simulink library "SOEM_EtherCAT_Lib"  (R2017b)
settings: Solver=ode45  StartTime=0.0  StopTime=10.0  RelTol=1e-3  EnableMultiTasking=on
settings Model: Creator=RecSet  LastModifiedBy=root
settings DataIOCC: LimitDataPoints=on  SaveFormat=Array
settings OptimizationCC: LifeSpan=inf
settings DebuggingCC: SolverPrmCheckMsg=warning  SFUnexpectedBacktrackingDiag=warning  SFNoUnconditionalDefaultTransitionDiag=warning  SFExecutionAtInitializationDiag=none
settings HardwareCC: ProdBitPerPointer=32  ProdBitPerSizeT=32  ProdBitPerPtrDiffT=32  ProdLargestAtomicFloat=None  ProdIntDivRoundTo=Undefined  ProdEndianess=Unspecified  ProdWordSize=32  ProdHWDeviceType=32-bit Generic
settings ModelReferenceCC: PropagateSignalLabelsOutOfModel=off
settings CodeAppCC: StateflowObjectComments=on
settings GRTTargetCC: TargetLangStandard=C89/C90 (ANSI)  GeneratePreprocessorConditionals=Disable all
settings ConfigComp: CovMetricSettings=dw  CovHtmlReporting=on  CovSaveCumulativeToWorkspaceVar=on  CovSaveSingleToWorkspaceVar=on  CovExternalEMLEnable=off  CovSFcnEnable=off

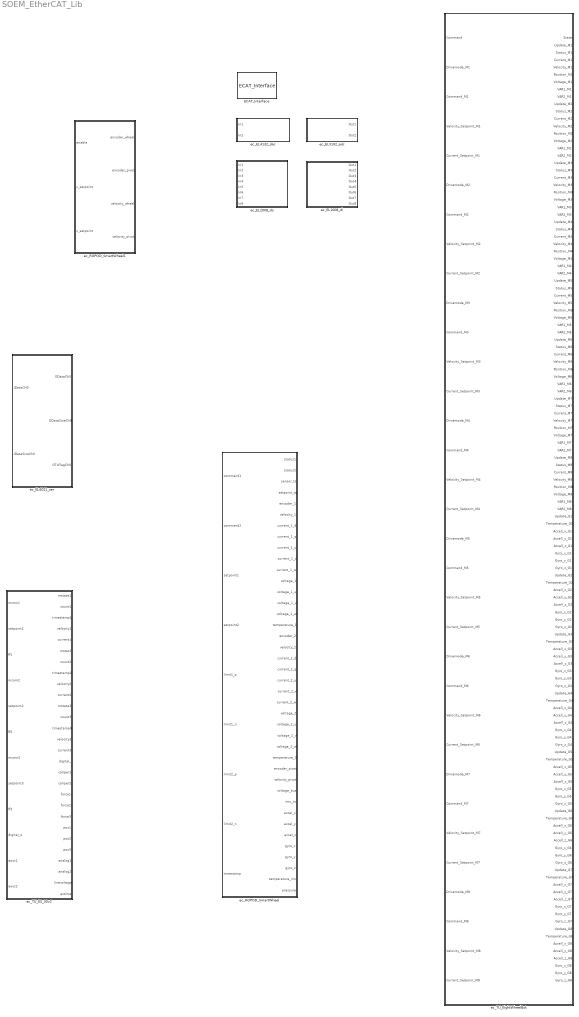
== system SOEM_EtherCAT_Lib ==
  ECAT_Interface : S-Function  Priority=0  StopFcn=|  FunctionName=ECAT_Interface  Parameters=IFINTERFACE,TS  SFunctionDeploymentMode=off  EnableBusSupport=off  mask{IFINTERFACE=eth0, TS=1/1000}
      | t_ = timer('Name','DLL_Unload_timer',...
      |             'ExecutionMode','singleShot',...
      |             'StartDelay',2,...
      |             'StopFcn','try;delete(t_);clear(''t_'');catch;disp(''Unloading DLL Failed!'');end;',...
      |             'TimerFcn','clear mex;'); 
      | start(t_);
      mask prompts: TS "Block sample time [s]"
      mask Callback IFINTERFACE:
      | VAR = get_param(gcb, 'IFINTERFACE');
      | if ~isnan(str2double(VAR))
      |     errordlg('Enter a string!');
      |     set_param(gcb, 'IFINTERFACE', '\Device\NPF_{$KEY}');
      | end
      mask DialogControl ParameterGroupVar Prompt: String with network device this block needs to use
  ec_EL1008_di : Subsystem  mask(EL1008 di){LINKID=1}
      mask prompts: LINKID "Enter link id (>0)"
  ec_EL2008_do : Subsystem  mask(EL2008 do){LINKID=1}
      mask prompts: LINKID "Enter link id (>0)"
  ec_EL3102_adc : Subsystem  mask(EL3102 adc){LINKID=1}
      mask prompts: LINKID "Enter link id (>0)"
  ec_EL4132_dac : Subsystem  mask(EL4132 dac){LINKID=1}
      mask prompts: LINKID "Enter link id (>0)"
  ec_EL6021_ser : Subsystem  mask{link_id=1}
      mask prompts: link_id "Link id (>0)"
  ec_ROPOD_SmartWheel : Subsystem  mask{link_id=1}
      mask prompts: link_id "Link id (>0)"
  ec_ROPOD_SmartWheel1 : Subsystem  mask{link_id=1}
      mask prompts: link_id "Link id (>0)"
  ec_TU_ES_30v2 : Subsystem  mask{link_id=1}
      mask prompts: link_id "Link id (>0)"
  ec_TU_EightWheelBot : Subsystem  mask(TU_EightWheelBot){LINKID=1}
      mask prompts: LINKID "Enter link id (>0)"

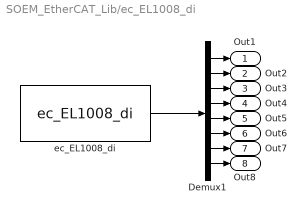
== system SOEM_EtherCAT_Lib/ec_EL1008_di ==
  Demux1 : Demux  Outputs=8
  ec_EL1008_di : S-Function  Priority=1  FunctionName=ec_EL1008_di  Parameters=LINKID  SFunctionDeploymentMode=off  EnableBusSupport=off
  Out1 : Outport
  Out2 : Outport  Port=2
  Out3 : Outport  Port=3
  Out4 : Outport  Port=4
  Out5 : Outport  Port=5
  Out6 : Outport  Port=6
  Out7 : Outport  Port=7
  Out8 : Outport  Port=8
  wires:
  Demux1/3 -> Out3/1
  Demux1/5 -> Out5/1
  Demux1/8 -> Out8/1
  Demux1/2 -> Out2/1
  Demux1/4 -> Out4/1
  Demux1/1 -> Out1/1
  Demux1/6 -> Out6/1
  Demux1/7 -> Out7/1
  ec_EL1008_di/1 -> Demux1/1

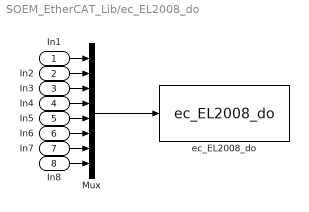
== system SOEM_EtherCAT_Lib/ec_EL2008_do ==
  In1 : Inport
  In2 : Inport  Port=2
  In3 : Inport  Port=3
  In4 : Inport  Port=4
  In5 : Inport  Port=5
  In6 : Inport  Port=6
  In7 : Inport  Port=7
  In8 : Inport  Port=8
  Mux : Mux  Inputs=8
  ec_EL2008_do : S-Function  Priority=1  FunctionName=ec_EL2008_do  Parameters=LINKID  SFunctionDeploymentMode=off  EnableBusSupport=off
  wires:
  In8/1 -> Mux/8
  In6/1 -> Mux/6
  In1/1 -> Mux/1
  In2/1 -> Mux/2
  In7/1 -> Mux/7
  In3/1 -> Mux/3
  In4/1 -> Mux/4
  In5/1 -> Mux/5
  Mux/1 -> ec_EL2008_do/1

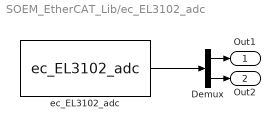
== system SOEM_EtherCAT_Lib/ec_EL3102_adc ==
  Demux : Demux  Outputs=2
  ec_EL3102_adc : S-Function  Priority=1  FunctionName=ec_EL3102_adc  Parameters=LINKID  SFunctionDeploymentMode=off  EnableBusSupport=off
  Out1 : Outport
  Out2 : Outport  Port=2
  wires:
  Demux/1 -> Out1/1
  Demux/2 -> Out2/1
  ec_EL3102_adc/1 -> Demux/1

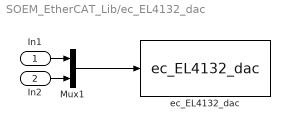
== system SOEM_EtherCAT_Lib/ec_EL4132_dac ==
  In1 : Inport
  In2 : Inport  Port=2
  Mux1 : Mux  Inputs=2
  ec_EL4132_dac : S-Function  Priority=1  FunctionName=ec_EL4132_dac  Parameters=LINKID  SFunctionDeploymentMode=off  EnableBusSupport=off
  wires:
  Mux1/1 -> ec_EL4132_dac/1
  In2/1 -> Mux1/2
  In1/1 -> Mux1/1

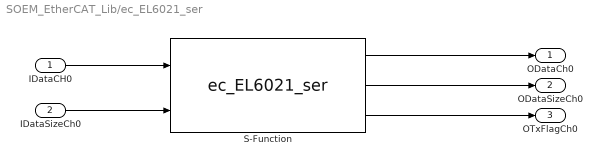
== system SOEM_EtherCAT_Lib/ec_EL6021_ser ==
  IDataCH0 : Inport
  IDataSizeCh0 : Inport  Port=2
  S-Function : S-Function  FunctionName=ec_EL6021_ser  Parameters=link_id  SFunctionDeploymentMode=off  EnableBusSupport=off  mask{link_id=link_id}
      mask prompts: link_id "Link id (start from 1)"
  ODataCh0 : Outport
  ODataSizeCh0 : Outport  Port=2
  OTxFlagCh0 : Outport  Port=3
  wires:
  IDataCH0/1 -> S-Function/1
  IDataSizeCh0/1 -> S-Function/2
  S-Function/1 -> ODataCh0/1
  S-Function/2 -> ODataSizeCh0/1
  S-Function/3 -> OTxFlagCh0/1

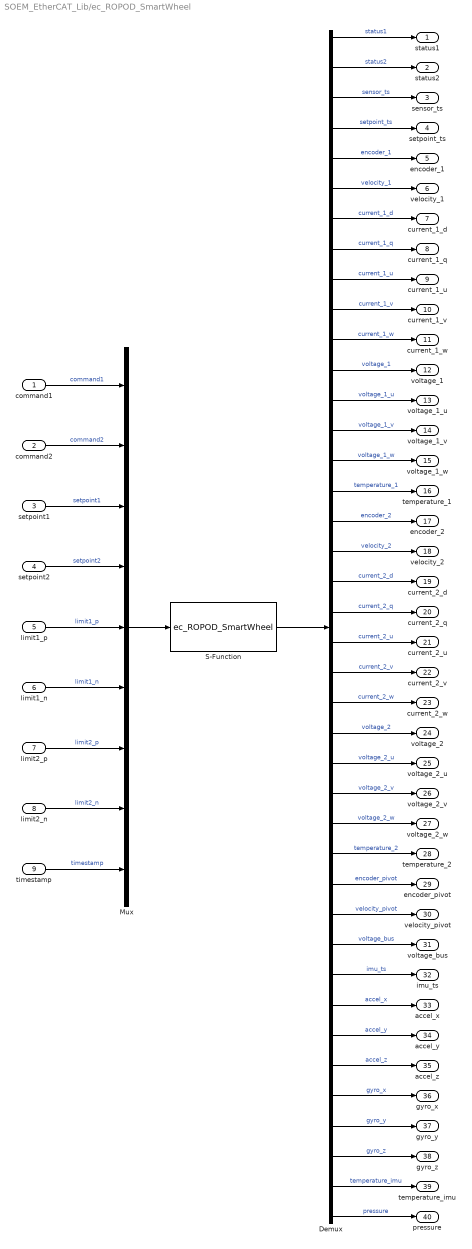
== system SOEM_EtherCAT_Lib/ec_ROPOD_SmartWheel ==
  command1 : Inport
  command2 : Inport  Port=2
  setpoint1 : Inport  Port=3
  setpoint2 : Inport  Port=4
  limit1_p : Inport  Port=5
  limit1_n : Inport  Port=6
  limit2_p : Inport  Port=7
  limit2_n : Inport  Port=8
  timestamp : Inport  Port=9
  Demux : Demux  Outputs=40
  Mux : Mux  Inputs=9
  S-Function : S-Function  FunctionName=ec_ROPOD_SmartWheel  Parameters=link_id  SFunctionDeploymentMode=off  EnableBusSupport=off  mask{link_id=link_id}
      mask prompts: link_id "Link id (start from 1)"
  status1 : Outport
  status2 : Outport  Port=2
  sensor_ts : Outport  Port=3
  setpoint_ts : Outport  Port=4
  encoder_1 : Outport  Port=5
  velocity_1 : Outport  Port=6
  current_1_d : Outport  Port=7
  current_1_q : Outport  Port=8
  current_1_u : Outport  Port=9
  current_1_v : Outport  Port=10
  current_1_w : Outport  Port=11
  voltage_1 : Outport  Port=12
  voltage_1_u : Outport  Port=13
  voltage_1_v : Outport  Port=14
  voltage_1_w : Outport  Port=15
  temperature_1 : Outport  Port=16
  encoder_2 : Outport  Port=17
  velocity_2 : Outport  Port=18
  current_2_d : Outport  Port=19
  current_2_q : Outport  Port=20
  current_2_u : Outport  Port=21
  current_2_v : Outport  Port=22
  current_2_w : Outport  Port=23
  voltage_2 : Outport  Port=24
  voltage_2_u : Outport  Port=25
  voltage_2_v : Outport  Port=26
  voltage_2_w : Outport  Port=27
  temperature_2 : Outport  Port=28
  encoder_pivot : Outport  Port=29
  velocity_pivot : Outport  Port=30
  voltage_bus : Outport  Port=31
  imu_ts : Outport  Port=32
  accel_x : Outport  Port=33
  accel_y : Outport  Port=34
  accel_z : Outport  Port=35
  gyro_x : Outport  Port=36
  gyro_y : Outport  Port=37
  gyro_z : Outport  Port=38
  temperature_imu : Outport  Port=39
  pressure : Outport  Port=40
  wires:
  Mux/1 -> S-Function/1
  timestamp/1 -> Mux/9  "timestamp"
  limit2_n/1 -> Mux/8  "limit2_n"
  limit2_p/1 -> Mux/7  "limit2_p"
  Demux/28 -> temperature_2/1  "temperature_2"
  Demux/27 -> voltage_2_w/1  "voltage_2_w"
  Demux/26 -> voltage_2_v/1  "voltage_2_v"
  Demux/25 -> voltage_2_u/1  "voltage_2_u"
  Demux/24 -> voltage_2/1  "voltage_2"
  Demux/23 -> current_2_w/1  "current_2_w"
  Demux/22 -> current_2_v/1  "current_2_v"
  Demux/21 -> current_2_u/1  "current_2_u"
  Demux/20 -> current_2_q/1  "current_2_q"
  Demux/19 -> current_2_d/1  "current_2_d"
  Demux/18 -> velocity_2/1  "velocity_2"
  Demux/17 -> encoder_2/1  "encoder_2"
  Demux/16 -> temperature_1/1  "temperature_1"
  Demux/15 -> voltage_1_w/1  "voltage_1_w"
  Demux/14 -> voltage_1_v/1  "voltage_1_v"
  Demux/13 -> voltage_1_u/1  "voltage_1_u"
  Demux/12 -> voltage_1/1  "voltage_1"
  Demux/11 -> current_1_w/1  "current_1_w"
  Demux/10 -> current_1_v/1  "current_1_v"
  Demux/9 -> current_1_u/1  "current_1_u"
  Demux/8 -> current_1_q/1  "current_1_q"
  Demux/7 -> current_1_d/1  "current_1_d"
  Demux/6 -> velocity_1/1  "velocity_1"
  Demux/5 -> encoder_1/1  "encoder_1"
  Demux/4 -> setpoint_ts/1  "setpoint_ts"
  Demux/3 -> sensor_ts/1  "sensor_ts"
  Demux/2 -> status2/1  "status2"
  limit1_n/1 -> Mux/6  "limit1_n"
  limit1_p/1 -> Mux/5  "limit1_p"
  setpoint2/1 -> Mux/4  "setpoint2"
  setpoint1/1 -> Mux/3  "setpoint1"
  Demux/1 -> status1/1  "status1"
  command2/1 -> Mux/2  "command2"
  command1/1 -> Mux/1  "command1"
  S-Function/1 -> Demux/1
  Demux/29 -> encoder_pivot/1  "encoder_pivot"
  Demux/30 -> velocity_pivot/1  "velocity_pivot"
  Demux/31 -> voltage_bus/1  "voltage_bus"
  Demux/32 -> imu_ts/1  "imu_ts"
  Demux/33 -> accel_x/1  "accel_x"
  Demux/34 -> accel_y/1  "accel_y"
  Demux/35 -> accel_z/1  "accel_z"
  Demux/36 -> gyro_x/1  "gyro_x"
  Demux/37 -> gyro_y/1  "gyro_y"
  Demux/38 -> gyro_z/1  "gyro_z"
  Demux/39 -> temperature_imu/1  "temperature_imu"
  Demux/40 -> pressure/1  "pressure"

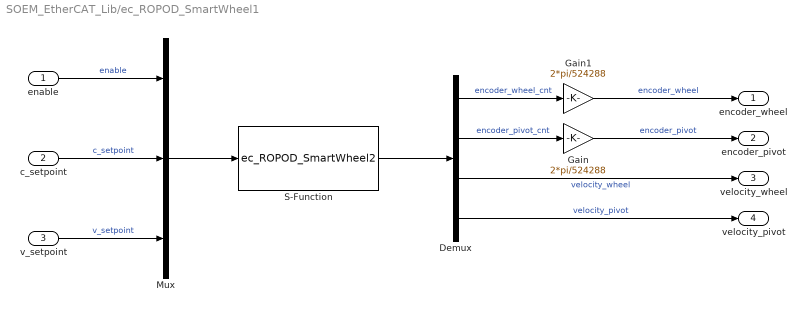
== system SOEM_EtherCAT_Lib/ec_ROPOD_SmartWheel1 ==
  enable : Inport
  c_setpoint : Inport  Port=2
  v_setpoint : Inport  Port=3
  Demux : Demux
  Gain : Gain  Gain=2*pi/524288
  Gain1 : Gain  Gain=2*pi/524288
  Mux : Mux  Inputs=3
  S-Function : S-Function  FunctionName=ec_ROPOD_SmartWheel2  Parameters=link_id  SFunctionDeploymentMode=off  EnableBusSupport=off  mask{link_id=link_id}
      mask prompts: link_id "Link id (start from 1)"
  encoder_wheel : Outport
  encoder_pivot : Outport  Port=2
  velocity_wheel : Outport  Port=3
  velocity_pivot : Outport  Port=4
  wires:
  Mux/1 -> S-Function/1
  Demux/4 -> velocity_pivot/1  "velocity_pivot"
  Demux/3 -> velocity_wheel/1  "velocity_wheel"
  Demux/2 -> Gain/1  "encoder_pivot_cnt"
  v_setpoint/1 -> Mux/3  "v_setpoint"
  Demux/1 -> Gain1/1  "encoder_wheel_cnt"
  c_setpoint/1 -> Mux/2  "c_setpoint"
  enable/1 -> Mux/1  "enable"
  S-Function/1 -> Demux/1
  Gain/1 -> encoder_pivot/1  "encoder_pivot"
  Gain1/1 -> encoder_wheel/1  "encoder_wheel"

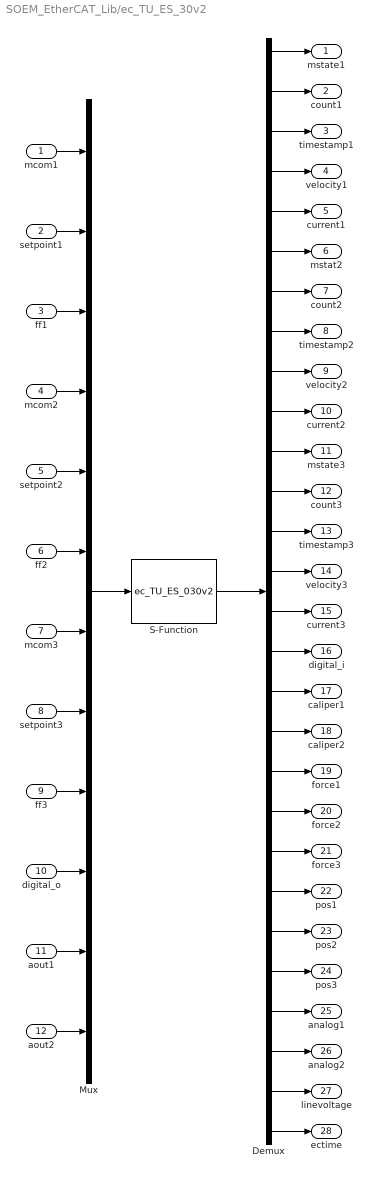
== system SOEM_EtherCAT_Lib/ec_TU_ES_30v2 ==
  mcom1 : Inport
  setpoint1 : Inport  Port=2
  ff1 : Inport  Port=3
  mcom2 : Inport  Port=4
  setpoint2 : Inport  Port=5
  ff2 : Inport  Port=6
  mcom3 : Inport  Port=7
  setpoint3 : Inport  Port=8
  ff3 : Inport  Port=9
  digital_o : Inport  Port=10
  aout1 : Inport  Port=11
  aout2 : Inport  Port=12
  Demux : Demux  Outputs=28
  Mux : Mux  Inputs=12
  S-Function : S-Function  FunctionName=ec_TU_ES_030v2  Parameters=link_id  SFunctionDeploymentMode=off  EnableBusSupport=off  mask{link_id=link_id}
      mask prompts: link_id "Link id (start from 1)"
  mstate1 : Outport
  count1 : Outport  Port=2
  timestamp1 : Outport  Port=3
  velocity1 : Outport  Port=4
  current1 : Outport  Port=5
  mstat2 : Outport  Port=6
  count2 : Outport  Port=7
  timestamp2 : Outport  Port=8
  velocity2 : Outport  Port=9
  current2 : Outport  Port=10
  mstate3 : Outport  Port=11
  count3 : Outport  Port=12
  timestamp3 : Outport  Port=13
  velocity3 : Outport  Port=14
  current3 : Outport  Port=15
  digital_i : Outport  Port=16
  caliper1 : Outport  Port=17
  caliper2 : Outport  Port=18
  force1 : Outport  Port=19
  force2 : Outport  Port=20
  force3 : Outport  Port=21
  pos1 : Outport  Port=22
  pos2 : Outport  Port=23
  pos3 : Outport  Port=24
  analog1 : Outport  Port=25
  analog2 : Outport  Port=26
  linevoltage : Outport  Port=27
  ectime : Outport  Port=28
  wires:
  S-Function/1 -> Demux/1
  mcom1/1 -> Mux/1
  setpoint1/1 -> Mux/2
  Demux/1 -> mstate1/1
  ff1/1 -> Mux/3
  mcom2/1 -> Mux/4
  setpoint2/1 -> Mux/5
  ff2/1 -> Mux/6
  Demux/2 -> count1/1
  Demux/3 -> timestamp1/1
  Demux/4 -> velocity1/1
  Demux/5 -> current1/1
  Demux/6 -> mstat2/1
  Demux/7 -> count2/1
  Demux/8 -> timestamp2/1
  Demux/9 -> velocity2/1
  Demux/10 -> current2/1
  Demux/11 -> mstate3/1
  Demux/12 -> count3/1
  Demux/13 -> timestamp3/1
  Demux/14 -> velocity3/1
  Demux/15 -> current3/1
  Demux/16 -> digital_i/1
  Demux/17 -> caliper1/1
  Demux/18 -> caliper2/1
  Demux/19 -> force1/1
  Demux/20 -> force2/1
  Demux/21 -> force3/1
  Demux/22 -> pos1/1
  Demux/23 -> pos2/1
  Demux/24 -> pos3/1
  Demux/25 -> analog1/1
  Demux/26 -> analog2/1
  Demux/27 -> linevoltage/1
  Demux/28 -> ectime/1
  mcom3/1 -> Mux/7
  setpoint3/1 -> Mux/8
  ff3/1 -> Mux/9
  digital_o/1 -> Mux/10
  aout1/1 -> Mux/11
  aout2/1 -> Mux/12
  Mux/1 -> S-Function/1

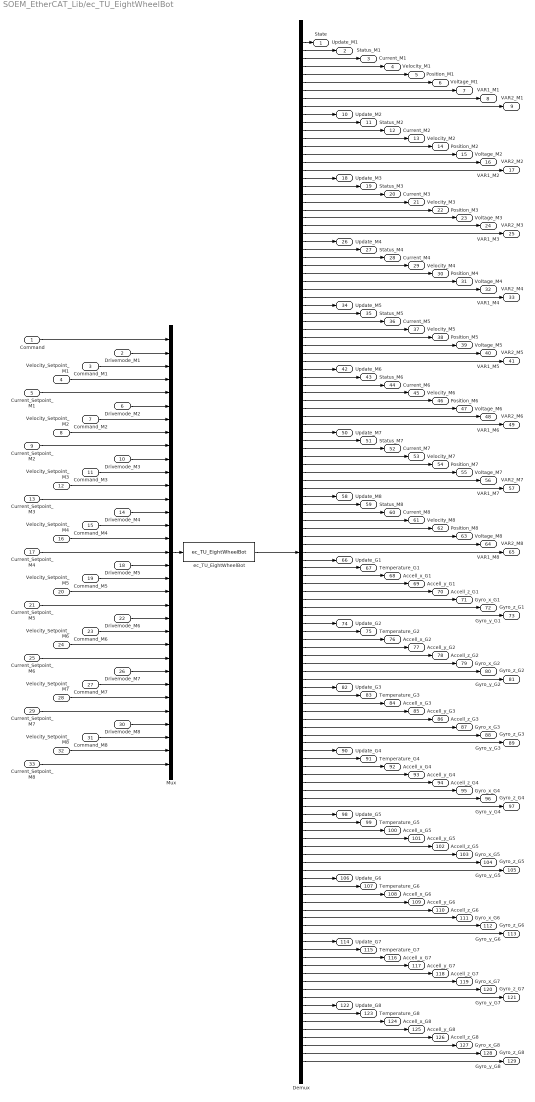
== system SOEM_EtherCAT_Lib/ec_TU_EightWheelBot ==
  Command : Inport
  Drivemode_M1 : Inport  Port=2
  Command_M1 : Inport  Port=3
  Velocity_Setpoint_M1 : Inport  Port=4
  Current_Setpoint_M1 : Inport  Port=5
  Drivemode_M2 : Inport  Port=6
  Command_M2 : Inport  Port=7
  Velocity_Setpoint_M2 : Inport  Port=8
  Current_Setpoint_M2 : Inport  Port=9
  Drivemode_M3 : Inport  Port=10
  Command_M3 : Inport  Port=11
  Velocity_Setpoint_M3 : Inport  Port=12
  Current_Setpoint_M3 : Inport  Port=13
  Drivemode_M4 : Inport  Port=14
  Command_M4 : Inport  Port=15
  Velocity_Setpoint_M4 : Inport  Port=16
  Current_Setpoint_M4 : Inport  Port=17
  Drivemode_M5 : Inport  Port=18
  Command_M5 : Inport  Port=19
  Velocity_Setpoint_M5 : Inport  Port=20
  Current_Setpoint_M5 : Inport  Port=21
  Drivemode_M6 : Inport  Port=22
  Command_M6 : Inport  Port=23
  Velocity_Setpoint_M6 : Inport  Port=24
  Current_Setpoint_M6 : Inport  Port=25
  Drivemode_M7 : Inport  Port=26
  Command_M7 : Inport  Port=27
  Velocity_Setpoint_M7 : Inport  Port=28
  Current_Setpoint_M7 : Inport  Port=29
  Drivemode_M8 : Inport  Port=30
  Command_M8 : Inport  Port=31
  Velocity_Setpoint_M8 : Inport  Port=32
  Current_Setpoint_M8 : Inport  Port=33
  Demux : Demux  Outputs=129
  Mux : Mux  Inputs=33
  ec_TU_EightWheelBot : S-Function  FunctionName=ec_TU_EightWheelBot  Parameters=LINKID  SFunctionDeploymentMode=off  EnableBusSupport=off
  State : Outport
  Update_M1 : Outport  Port=2
  Status_M1 : Outport  Port=3
  Current_M1 : Outport  Port=4
  Velocity_M1 : Outport  Port=5
  Position_M1 : Outport  Port=6
  Voltage_M1 : Outport  Port=7
  VAR1_M1 : Outport  Port=8
  VAR2_M1 : Outport  Port=9
  Update_M2 : Outport  Port=10
  Status_M2 : Outport  Port=11
  Current_M2 : Outport  Port=12
  Velocity_M2 : Outport  Port=13
  Position_M2 : Outport  Port=14
  Voltage_M2 : Outport  Port=15
  VAR1_M2 : Outport  Port=16
  VAR2_M2 : Outport  Port=17
  Update_M3 : Outport  Port=18
  Status_M3 : Outport  Port=19
  Current_M3 : Outport  Port=20
  Velocity_M3 : Outport  Port=21
  Position_M3 : Outport  Port=22
  Voltage_M3 : Outport  Port=23
  VAR1_M3 : Outport  Port=24
  VAR2_M3 : Outport  Port=25
  Update_M4 : Outport  Port=26
  Status_M4 : Outport  Port=27
  Current_M4 : Outport  Port=28
  Velocity_M4 : Outport  Port=29
  Position_M4 : Outport  Port=30
  Voltage_M4 : Outport  Port=31
  VAR1_M4 : Outport  Port=32
  VAR2_M4 : Outport  Port=33
  Update_M5 : Outport  Port=34
  Status_M5 : Outport  Port=35
  Current_M5 : Outport  Port=36
  Velocity_M5 : Outport  Port=37
  Position_M5 : Outport  Port=38
  Voltage_M5 : Outport  Port=39
  VAR1_M5 : Outport  Port=40
  VAR2_M5 : Outport  Port=41
  Update_M6 : Outport  Port=42
  Status_M6 : Outport  Port=43
  Current_M6 : Outport  Port=44
  Velocity_M6 : Outport  Port=45
  Position_M6 : Outport  Port=46
  Voltage_M6 : Outport  Port=47
  VAR1_M6 : Outport  Port=48
  VAR2_M6 : Outport  Port=49
  Update_M7 : Outport  Port=50
  Status_M7 : Outport  Port=51
  Current_M7 : Outport  Port=52
  Velocity_M7 : Outport  Port=53
  Position_M7 : Outport  Port=54
  Voltage_M7 : Outport  Port=55
  VAR1_M7 : Outport  Port=56
  VAR2_M7 : Outport  Port=57
  Update_M8 : Outport  Port=58
  Status_M8 : Outport  Port=59
  Current_M8 : Outport  Port=60
  Velocity_M8 : Outport  Port=61
  Position_M8 : Outport  Port=62
  Voltage_M8 : Outport  Port=63
  VAR1_M8 : Outport  Port=64
  VAR2_M8 : Outport  Port=65
  Update_G1 : Outport  Port=66
  Temperature_G1 : Outport  Port=67
  Accell_x_G1 : Outport  Port=68
  Accell_y_G1 : Outport  Port=69
  Accell_z_G1 : Outport  Port=70
  Gyro_x_G1 : Outport  Port=71
  Gyro_y_G1 : Outport  Port=72
  Gyro_z_G1 : Outport  Port=73
  Update_G2 : Outport  Port=74
  Temperature_G2 : Outport  Port=75
  Accell_x_G2 : Outport  Port=76
  Accell_y_G2 : Outport  Port=77
  Accell_z_G2 : Outport  Port=78
  Gyro_x_G2 : Outport  Port=79
  Gyro_y_G2 : Outport  Port=80
  Gyro_z_G2 : Outport  Port=81
  Update_G3 : Outport  Port=82
  Temperature_G3 : Outport  Port=83
  Accell_x_G3 : Outport  Port=84
  Accell_y_G3 : Outport  Port=85
  Accell_z_G3 : Outport  Port=86
  Gyro_x_G3 : Outport  Port=87
  Gyro_y_G3 : Outport  Port=88
  Gyro_z_G3 : Outport  Port=89
  Update_G4 : Outport  Port=90
  Temperature_G4 : Outport  Port=91
  Accell_x_G4 : Outport  Port=92
  Accell_y_G4 : Outport  Port=93
  Accell_z_G4 : Outport  Port=94
  Gyro_x_G4 : Outport  Port=95
  Gyro_y_G4 : Outport  Port=96
  Gyro_z_G4 : Outport  Port=97
  Update_G5 : Outport  Port=98
  Temperature_G5 : Outport  Port=99
  Accell_x_G5 : Outport  Port=100
  Accell_y_G5 : Outport  Port=101
  Accell_z_G5 : Outport  Port=102
  Gyro_x_G5 : Outport  Port=103
  Gyro_y_G5 : Outport  Port=104
  Gyro_z_G5 : Outport  Port=105
  Update_G6 : Outport  Port=106
  Temperature_G6 : Outport  Port=107
  Accell_x_G6 : Outport  Port=108
  Accell_y_G6 : Outport  Port=109
  Accell_z_G6 : Outport  Port=110
  Gyro_x_G6 : Outport  Port=111
  Gyro_y_G6 : Outport  Port=112
  Gyro_z_G6 : Outport  Port=113
  Update_G7 : Outport  Port=114
  Temperature_G7 : Outport  Port=115
  Accell_x_G7 : Outport  Port=116
  Accell_y_G7 : Outport  Port=117
  Accell_z_G7 : Outport  Port=118
  Gyro_x_G7 : Outport  Port=119
  Gyro_y_G7 : Outport  Port=120
  Gyro_z_G7 : Outport  Port=121
  Update_G8 : Outport  Port=122
  Temperature_G8 : Outport  Port=123
  Accell_x_G8 : Outport  Port=124
  Accell_y_G8 : Outport  Port=125
  Accell_z_G8 : Outport  Port=126
  Gyro_x_G8 : Outport  Port=127
  Gyro_y_G8 : Outport  Port=128
  Gyro_z_G8 : Outport  Port=129
  wires:
  ec_TU_EightWheelBot/1 -> Demux/1
  Command/1 -> Mux/1
  Mux/1 -> ec_TU_EightWheelBot/1
  Demux/1 -> State/1
  Demux/2 -> Update_M1/1
  Demux/3 -> Status_M1/1
  Demux/9 -> VAR2_M1/1
  Demux/8 -> VAR1_M1/1
  Demux/7 -> Voltage_M1/1
  Demux/6 -> Position_M1/1
  Demux/5 -> Velocity_M1/1
  Demux/4 -> Current_M1/1
  Demux/10 -> Update_M2/1
  Demux/11 -> Status_M2/1
  Demux/17 -> VAR2_M2/1
  Demux/16 -> VAR1_M2/1
  Demux/15 -> Voltage_M2/1
  Demux/14 -> Position_M2/1
  Demux/13 -> Velocity_M2/1
  Demux/12 -> Current_M2/1
  Demux/18 -> Update_M3/1
  Demux/19 -> Status_M3/1
  Demux/25 -> VAR2_M3/1
  Demux/24 -> VAR1_M3/1
  Demux/23 -> Voltage_M3/1
  Demux/22 -> Position_M3/1
  Demux/21 -> Velocity_M3/1
  Demux/20 -> Current_M3/1
  Demux/26 -> Update_M4/1
  Demux/27 -> Status_M4/1
  Demux/33 -> VAR2_M4/1
  Demux/32 -> VAR1_M4/1
  Demux/31 -> Voltage_M4/1
  Demux/30 -> Position_M4/1
  Demux/29 -> Velocity_M4/1
  Demux/28 -> Current_M4/1
  Demux/34 -> Update_M5/1
  Demux/35 -> Status_M5/1
  Demux/41 -> VAR2_M5/1
  Demux/40 -> VAR1_M5/1
  Demux/39 -> Voltage_M5/1
  Demux/38 -> Position_M5/1
  Demux/37 -> Velocity_M5/1
  Demux/36 -> Current_M5/1
  Demux/42 -> Update_M6/1
  Demux/43 -> Status_M6/1
  Demux/49 -> VAR2_M6/1
  Demux/48 -> VAR1_M6/1
  Demux/47 -> Voltage_M6/1
  Demux/46 -> Position_M6/1
  Demux/45 -> Velocity_M6/1
  Demux/44 -> Current_M6/1
  Demux/50 -> Update_M7/1
  Demux/51 -> Status_M7/1
  Demux/57 -> VAR2_M7/1
  Demux/56 -> VAR1_M7/1
  Demux/55 -> Voltage_M7/1
  Demux/54 -> Position_M7/1
  Demux/53 -> Velocity_M7/1
  Demux/52 -> Current_M7/1
  Demux/58 -> Update_M8/1
  Demux/59 -> Status_M8/1
  Demux/65 -> VAR2_M8/1
  Demux/64 -> VAR1_M8/1
  Demux/63 -> Voltage_M8/1
  Demux/62 -> Position_M8/1
  Demux/61 -> Velocity_M8/1
  Demux/60 -> Current_M8/1
  Demux/66 -> Update_G1/1
  Demux/67 -> Temperature_G1/1
  Demux/73 -> Gyro_z_G1/1
  Demux/72 -> Gyro_y_G1/1
  Demux/71 -> Gyro_x_G1/1
  Demux/70 -> Accell_z_G1/1
  Demux/69 -> Accell_y_G1/1
  Demux/68 -> Accell_x_G1/1
  Demux/74 -> Update_G2/1
  Demux/75 -> Temperature_G2/1
  Demux/81 -> Gyro_z_G2/1
  Demux/80 -> Gyro_y_G2/1
  Demux/79 -> Gyro_x_G2/1
  Demux/78 -> Accell_z_G2/1
  Demux/77 -> Accell_y_G2/1
  Demux/76 -> Accell_x_G2/1
  Demux/82 -> Update_G3/1
  Demux/83 -> Temperature_G3/1
  Demux/89 -> Gyro_z_G3/1
  Demux/88 -> Gyro_y_G3/1
  Demux/87 -> Gyro_x_G3/1
  Demux/86 -> Accell_z_G3/1
  Demux/85 -> Accell_y_G3/1
  Demux/84 -> Accell_x_G3/1
  Demux/90 -> Update_G4/1
  Demux/91 -> Temperature_G4/1
  Demux/97 -> Gyro_z_G4/1
  Demux/96 -> Gyro_y_G4/1
  Demux/95 -> Gyro_x_G4/1
  Demux/94 -> Accell_z_G4/1
  Demux/93 -> Accell_y_G4/1
  Demux/92 -> Accell_x_G4/1
  Demux/98 -> Update_G5/1
  Demux/99 -> Temperature_G5/1
  Demux/105 -> Gyro_z_G5/1
  Demux/104 -> Gyro_y_G5/1
  Demux/103 -> Gyro_x_G5/1
  Demux/102 -> Accell_z_G5/1
  Demux/101 -> Accell_y_G5/1
  Demux/100 -> Accell_x_G5/1
  Demux/106 -> Update_G6/1
  Demux/107 -> Temperature_G6/1
  Demux/113 -> Gyro_z_G6/1
  Demux/112 -> Gyro_y_G6/1
  Demux/111 -> Gyro_x_G6/1
  Demux/110 -> Accell_z_G6/1
  Demux/109 -> Accell_y_G6/1
  Demux/108 -> Accell_x_G6/1
  Demux/114 -> Update_G7/1
  Demux/115 -> Temperature_G7/1
  Demux/121 -> Gyro_z_G7/1
  Demux/120 -> Gyro_y_G7/1
  Demux/119 -> Gyro_x_G7/1
  Demux/118 -> Accell_z_G7/1
  Demux/117 -> Accell_y_G7/1
  Demux/116 -> Accell_x_G7/1
  Demux/122 -> Update_G8/1
  Demux/123 -> Temperature_G8/1
  Demux/129 -> Gyro_z_G8/1
  Demux/128 -> Gyro_y_G8/1
  Demux/127 -> Gyro_x_G8/1
  Demux/126 -> Accell_z_G8/1
  Demux/125 -> Accell_y_G8/1
  Demux/124 -> Accell_x_G8/1
  Drivemode_M1/1 -> Mux/2
  Command_M1/1 -> Mux/3
  Velocity_Setpoint_M1/1 -> Mux/4
  Current_Setpoint_M1/1 -> Mux/5
  Drivemode_M2/1 -> Mux/6
  Command_M2/1 -> Mux/7
  Velocity_Setpoint_M2/1 -> Mux/8
  Current_Setpoint_M2/1 -> Mux/9
  Drivemode_M3/1 -> Mux/10
  Command_M3/1 -> Mux/11
  Velocity_Setpoint_M3/1 -> Mux/12
  Current_Setpoint_M3/1 -> Mux/13
  Drivemode_M4/1 -> Mux/14
  Command_M4/1 -> Mux/15
  Velocity_Setpoint_M4/1 -> Mux/16
  Current_Setpoint_M4/1 -> Mux/17
  Drivemode_M5/1 -> Mux/18
  Command_M5/1 -> Mux/19
  Velocity_Setpoint_M5/1 -> Mux/20
  Current_Setpoint_M5/1 -> Mux/21
  Drivemode_M6/1 -> Mux/22
  Command_M6/1 -> Mux/23
  Velocity_Setpoint_M6/1 -> Mux/24
  Current_Setpoint_M6/1 -> Mux/25
  Drivemode_M7/1 -> Mux/26
  Command_M7/1 -> Mux/27
  Velocity_Setpoint_M7/1 -> Mux/28
  Current_Setpoint_M7/1 -> Mux/29
  Drivemode_M8/1 -> Mux/30
  Command_M8/1 -> Mux/31
  Velocity_Setpoint_M8/1 -> Mux/32
  Current_Setpoint_M8/1 -> Mux/33
